simulink subsystem "subref_mix_yaw"  (R2024b)
settings: Solver=VariableStepAuto  StartTime=0.0  StopTime=10.0  RelTol=1e-3
settings Model: Creator=CETCA  LastModifiedBy=CETCA

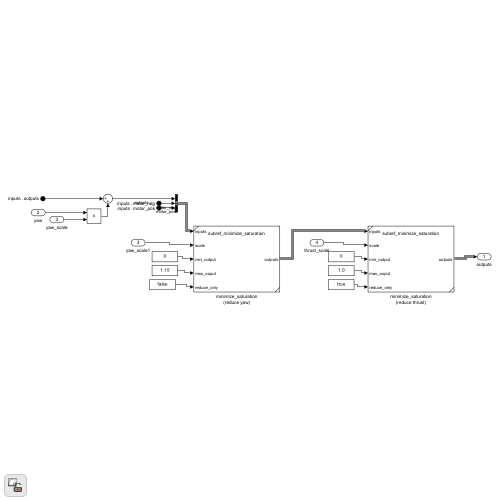
[thumbnail: Simulink's stored preview of the top-level diagram]
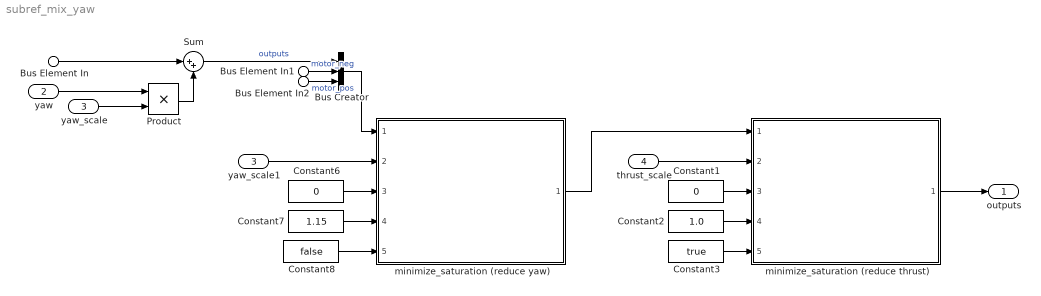
== system subref_mix_yaw ==
  Bus Element In : Inport  PortName=inputs  Element=outputs
  Bus Element In1 : Inport  PortName=inputs  Element=motor_neg
  Bus Element In2 : Inport  PortName=inputs  Element=motor_pos
  yaw : Inport  Port=2
  yaw_scale : Inport  Port=3
  thrust_scale : Inport  Port=4
  Bus Creator : BusCreator  Inputs=3
  Constant1 : Constant  Value=0
  Constant2 : Constant  Value=1.0
  Constant3 : Constant  Value=true
  Constant6 : Constant  Value=0
  Constant7 : Constant  Value=1.15
  Constant8 : Constant  Value=false
  Product : Product
  Sum : Sum  Inputs=|++
  minimize_saturation (reduce thrust) : Subsystem  ReferencedSubsystem=subref_minimize_saturation
  minimize_saturation (reduce yaw) : Subsystem  ReferencedSubsystem=subref_minimize_saturation
  yaw_scale1 : InportShadow  Port=3
  outputs : Outport
  wires:
  Bus Element In/1 -> Sum/1
  yaw/1 -> Product/1
  yaw_scale/1 -> Product/2
  Product/1 -> Sum/2
  Constant6/1 -> minimize_saturation (reduce yaw)/3
  Constant7/1 -> minimize_saturation (reduce yaw)/4
  Constant8/1 -> minimize_saturation (reduce yaw)/5
  thrust_scale/1 -> minimize_saturation (reduce thrust)/2
  minimize_saturation (reduce yaw)/1 -> minimize_saturation (reduce thrust)/1
  Constant1/1 -> minimize_saturation (reduce thrust)/3
  Constant2/1 -> minimize_saturation (reduce thrust)/4
  Constant3/1 -> minimize_saturation (reduce thrust)/5
  minimize_saturation (reduce thrust)/1 -> outputs/1
  yaw_scale1/1 -> minimize_saturation (reduce yaw)/2
  Sum/1 -> Bus Creator/1  "outputs"
  Bus Creator/1 -> minimize_saturation (reduce yaw)/1
  Bus Element In1/1 -> Bus Creator/2  "motor_neg"
  Bus Element In2/1 -> Bus Creator/3  "motor_pos"
